simulink model "test03_mod04"  (Simulink 7.3)
settings: Solver=FixedStepDiscrete  SolverMode=SingleTasking  StartTime=0.0  StopTime=inf  FixedStep=0.01  RelTol=1e-3  SampleTimeConstraint=Specified
undefined symbols (not defined in the file or in its folder): serial
libraries: simulink x5, instrumentlib x2
settings Model: Creator=Administrateur  LastModifiedBy=Administrateur
settings MATStruct: SampleTime=0.1  Offset=0  Priority=[10.0]

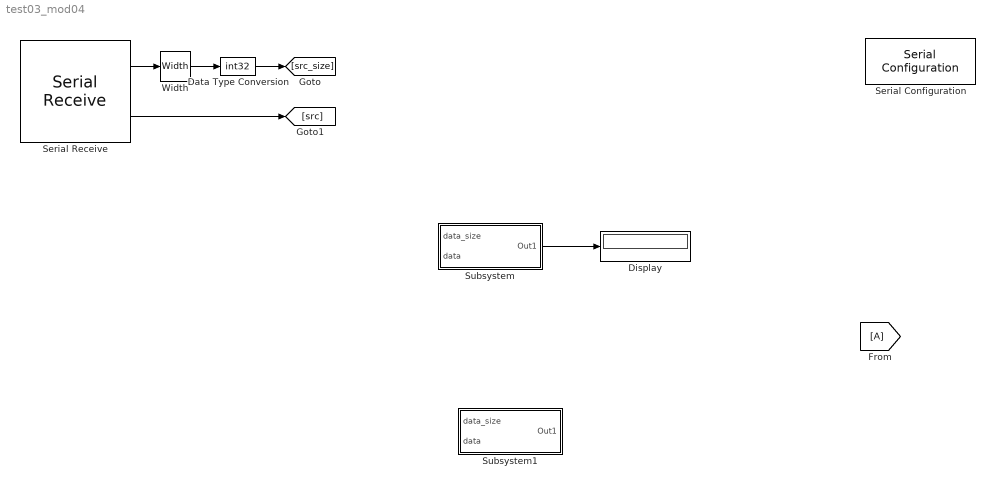
== system test03_mod04 ==
  Data Type Conversion : DataTypeConversion  OutDataTypeMode=int32  OutDataType=fixdt(1, 16)  OutScaling=2^0  OutDataTypeStr=int32
  Display : Display
  Serial Configuration : instrumentlib/Serial Configuration  Priority=-200000  DialogController=instrumentcreatedialog  DialogControllerArgs=DataTag0  ComPortMenu=COM4  ComPort=COM4  ObjConstructor=serial('COM4');  BaudRate=38400  DataBits=8  Parity=none  StopBits=1  FlowControl=none  Timeout=10  ByteOrder=LittleEndian
  Serial Receive : instrumentlib/Serial Receive  DialogController=instrumentcreatedialog  DialogControllerArgs=DataTag1  ComPortMenu=COM4  ComPort=COM4  ObjConstructor=serial('COM4');  Terminator=<none>  DataSize="[40   1]"  DataType=uint8  EnableBlockingMode=off  ActionDataUnavailable=Output last received value  CustomValue=0  SampleTime=-1
  Subsystem : Subsystem
  Subsystem1 : Subsystem
  Width : Width
  wires:
  Width/1 -> Data Type Conversion/1
  Subsystem/1(Out1) -> Display/1
  Data Type Conversion/1 -> [src_size]
  Serial Receive/1 -> Width/1
  Serial Receive/2 -> [src]

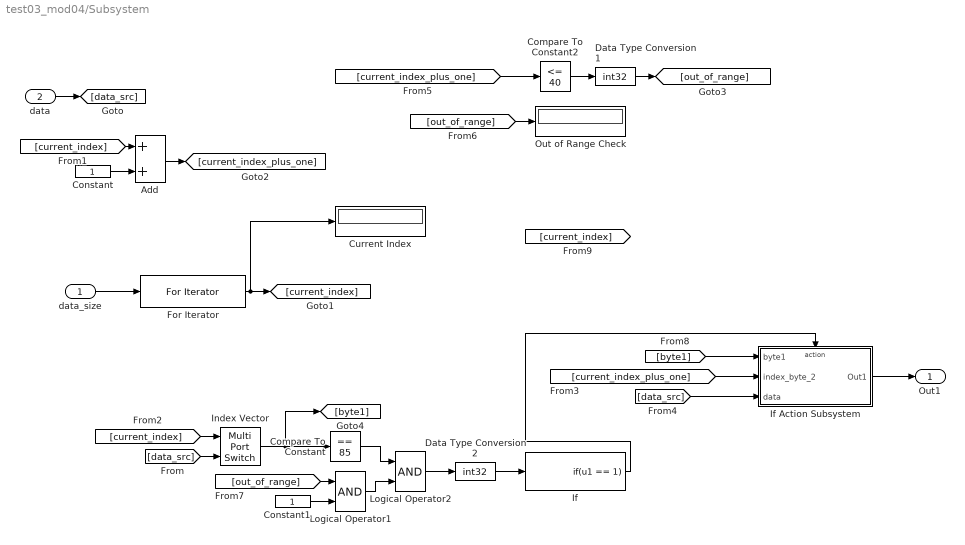
== system test03_mod04/Subsystem ==
  data_size : Inport  DataType=int32  OutDataType=fixdt(1, 16)  OutScaling=2^0  OutDataTypeStr=int32
  data : Inport  Port=2  DataType=uint8  OutDataType=fixdt(1, 16)  OutScaling=2^0  OutDataTypeStr=uint8
  Add : Sum  AccumDataTypeStr=int32  OutDataTypeMode=int32  OutDataType=fixdt(1, 16)  OutScaling=2^-10  OutDataTypeStr=int32
  Compare To Constant : simulink/Logic and Bit Operations/Compare To Constant  SystemSampleTime=-1  relop===  const=85  LogicOutDataTypeMode=uint8  ZeroCross=off
  Compare To Constant2 : simulink/Logic and Bit Operations/Compare To Constant  SystemSampleTime=-1  relop=<=  const=40  LogicOutDataTypeMode=boolean  ZeroCross=off
  Constant : Constant  OutDataTypeMode=int32  OutDataType=fixdt(1, 16)  OutScaling=2^0  OutDataTypeStr=int32  SampleTime=-1
  Constant1 : Constant  OutDataTypeMode=int32  OutDataType=fixdt(1, 16)  OutScaling=2^0  OutDataTypeStr=int32  SampleTime=-1
  Current Index : Display
  Data Type Conversion1 : DataTypeConversion  OutDataTypeMode=int32  OutDataType=fixdt(1, 16)  OutScaling=2^0  OutDataTypeStr=int32
  Data Type Conversion2 : DataTypeConversion  OutDataTypeMode=int32  OutDataType=fixdt(1, 16)  OutScaling=2^0  OutDataTypeStr=int32
  For Iterator : ForIterator  IterationSource=external
  If : If  IfExpression=u1 == 1  ShowElse=off
  If Action Subsystem : Subsystem  TreatAsAtomicUnit=on
  Index Vector : MultiPortSwitch  Inputs=1  zeroidx=on  OutDataType=fixdt(1, 16)  OutScaling=2^0
  Logical Operator1 : Logic  AllPortsSameDT=off  OutDataTypeMode=boolean  LogicDataType=fixdt(0, 8)  OutDataTypeStr=boolean
  Logical Operator2 : Logic  AllPortsSameDT=off  OutDataTypeMode=boolean  LogicDataType=fixdt(0, 8)  OutDataTypeStr=boolean
  Out of Range Check : Display
  Out1 : Outport  DataType=boolean  OutDataType=fixdt(1, 16)  OutScaling=2^0  OutDataTypeStr=boolean
  wires:
  data_size/1 -> For Iterator/1
  data/1 -> [data_src]
  [data_src] -> Index Vector/2
  For Iterator/1 -> [current_index], Current Index/1
  Constant/1 -> Add/2
  [current_index] -> Add/1
  Add/1 -> [current_index_plus_one]
  [current_index] -> Index Vector/1
  Index Vector/1 -> Compare To Constant/1, [byte1]
  [current_index_plus_one] -> Compare To Constant2/1
  Compare To Constant2/1 -> Data Type Conversion1/1
  Data Type Conversion1/1 -> [out_of_range]
  [out_of_range] -> Out of Range Check/1
  [out_of_range] -> Logical Operator1/1
  Constant1/1 -> Logical Operator1/2
  Logical Operator1/1 -> Logical Operator2/2
  Compare To Constant/1 -> Logical Operator2/1
  Logical Operator2/1 -> Data Type Conversion2/1
  Data Type Conversion2/1 -> If/1
  [byte1] -> If Action Subsystem/1(byte1)
  [current_index_plus_one] -> If Action Subsystem/2(index_byte_2)
  [data_src] -> If Action Subsystem/3(data)
  If/1 -> If Action Subsystem/Action
  If Action Subsystem/1(Out1) -> Out1/1

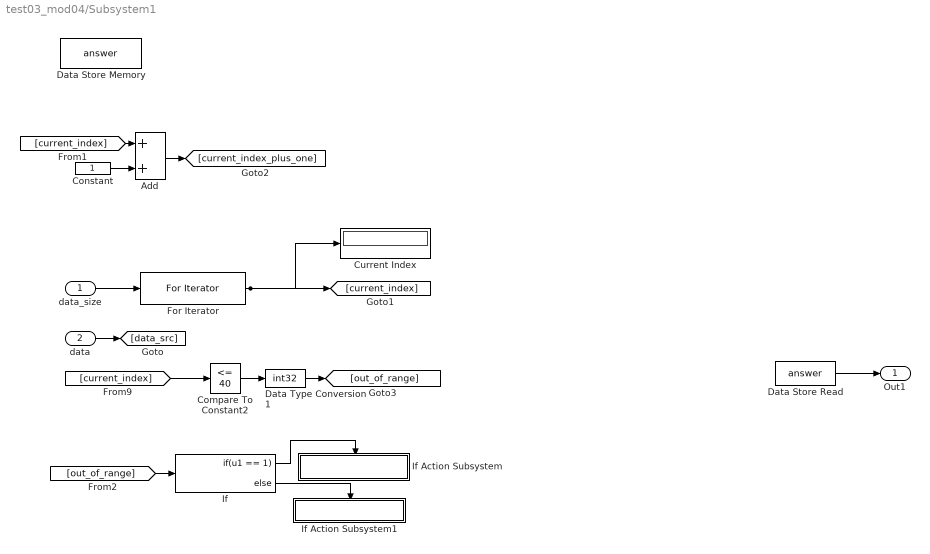
== system test03_mod04/Subsystem1 ==
  data_size : Inport  DataType=int32  OutDataType=fixdt(1, 16)  OutScaling=2^0  OutDataTypeStr=int32
  data : Inport  Port=2  DataType=uint8  OutDataType=fixdt(1, 16)  OutScaling=2^0  OutDataTypeStr=uint8
  Add : Sum  AccumDataTypeStr=int32  OutDataTypeMode=int32  OutDataType=fixdt(1, 16)  OutScaling=2^-10  OutDataTypeStr=int32
  Compare To Constant2 : simulink/Logic and Bit Operations/Compare To Constant  SystemSampleTime=-1  relop=<=  const=40  LogicOutDataTypeMode=boolean  ZeroCross=off
  Constant : Constant  OutDataTypeMode=int32  OutDataType=fixdt(1, 16)  OutScaling=2^0  OutDataTypeStr=int32  SampleTime=-1
  Current Index : Display
  Data Store Memory : DataStoreMemory  DataStoreName=answer  DataType=int32  OutDataType=fixdt(1, 16)  OutScaling=2^0  OutDataTypeStr=int32
  Data Store Read : DataStoreRead  DataStoreName=answer  SampleTime=-1
  Data Type Conversion1 : DataTypeConversion  OutDataTypeMode=int32  OutDataType=fixdt(1, 16)  OutScaling=2^0  OutDataTypeStr=int32
  For Iterator : ForIterator  IterationSource=external
  If : If  IfExpression=u1 == 1
  If Action Subsystem : Subsystem  TreatAsAtomicUnit=on
  If Action Subsystem1 : Subsystem  TreatAsAtomicUnit=on
  Out1 : Outport  DataType=int32  OutDataType=fixdt(1, 16)  OutScaling=2^0  OutDataTypeStr=int32
  wires:
  data_size/1 -> For Iterator/1
  data/1 -> [data_src]
  For Iterator/1 -> [current_index], Current Index/1
  Constant/1 -> Add/2
  [current_index] -> Add/1
  Add/1 -> [current_index_plus_one]
  Compare To Constant2/1 -> Data Type Conversion1/1
  Data Type Conversion1/1 -> [out_of_range]
  [current_index] -> Compare To Constant2/1
  [out_of_range] -> If/1
  If/2 -> If Action Subsystem1/Action
  If/1 -> If Action Subsystem/Action
  Data Store Read/1 -> Out1/1

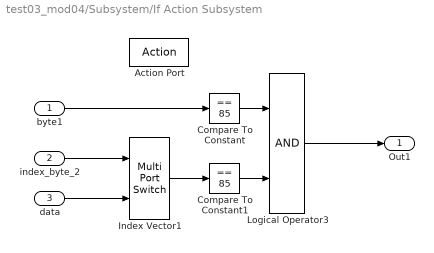
== system test03_mod04/Subsystem/If Action Subsystem ==
  byte1 : Inport  DataType=uint8  OutDataType=fixdt(1, 16)  OutScaling=2^0  OutDataTypeStr=uint8
  index_byte_2 : Inport  Port=2  DataType=int32  OutDataType=fixdt(1, 16)  OutScaling=2^0  OutDataTypeStr=int32
  data : Inport  Port=3  DataType=uint8  OutDataType=fixdt(1, 16)  OutScaling=2^0  OutDataTypeStr=uint8
  Action Port : ActionPort  ActionType=then
  Compare To Constant : simulink/Logic and Bit Operations/Compare To Constant  SystemSampleTime=-1  relop===  const=85  LogicOutDataTypeMode=uint8  ZeroCross=off
  Compare To Constant1 : simulink/Logic and Bit Operations/Compare To Constant  SystemSampleTime=-1  relop===  const=85  LogicOutDataTypeMode=uint8  ZeroCross=off
  Index Vector1 : MultiPortSwitch  Inputs=1  zeroidx=on  OutDataType=fixdt(1, 16)  OutScaling=2^0
  Logical Operator3 : Logic  AllPortsSameDT=off  OutDataTypeMode=boolean  LogicDataType=fixdt(0, 8)  OutDataTypeStr=boolean
  Out1 : Outport  DataType=boolean  OutDataType=fixdt(1, 16)  OutScaling=2^0  OutDataTypeStr=boolean  InitialOutput=[0]
  wires:
  Index Vector1/1 -> Compare To Constant1/1
  data/1 -> Index Vector1/2
  index_byte_2/1 -> Index Vector1/1
  byte1/1 -> Compare To Constant/1
  Compare To Constant1/1 -> Logical Operator3/2
  Compare To Constant/1 -> Logical Operator3/1
  Logical Operator3/1 -> Out1/1

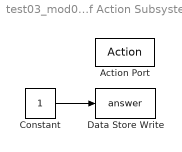
== system test03_mod04/Subsystem1/If Action Subsystem ==
  Action Port : ActionPort  ActionType=then
  Constant : Constant  OutDataTypeMode=int32  OutDataType=fixdt(1, 16)  OutScaling=2^0  OutDataTypeStr=int32  SampleTime=-1
  Data Store Write : DataStoreWrite  DataStoreName=answer  SampleTime=-1
  wires:
  Constant/1 -> Data Store Write/1

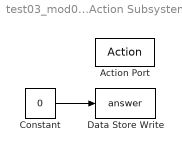
== system test03_mod04/Subsystem1/If Action Subsystem1 ==
  Action Port : ActionPort  ActionType=else
  Constant : Constant  Value=0  OutDataTypeMode=int32  OutDataType=fixdt(1, 16)  OutScaling=2^0  OutDataTypeStr=int32  SampleTime=-1
  Data Store Write : DataStoreWrite  DataStoreName=answer  SampleTime=-1
  wires:
  Constant/1 -> Data Store Write/1
